simulink model "SF003A_Dampg"  (R2013b)
settings: Solver=FixedStepDiscrete  StartTime=0.0  StopTime=1  FixedStep=.002  RelTol=1e-3
values from neighbouring files (symbols this model uses):
  ARCHGLBPRM_2MILLISEC_SEC_F32 = DataDict.Constant    [SF003A_Dampg_DataDict.m]
  DampgHydBasCoeff1 = DataDict.Calibration    [SF003A_Dampg_DataDict.m]
  DampgHydBasCoeff2 = DataDict.Calibration    [SF003A_Dampg_DataDict.m]
  DampgHydBasCoeff3 = DataDict.Calibration    [SF003A_Dampg_DataDict.m]
  DampgHydBasCoeff4 = DataDict.Calibration    [SF003A_Dampg_DataDict.m]
  DampgHydOutpLim = DataDict.Calibration    [SF003A_Dampg_DataDict.m]
  DampgQuad13Mplr = DataDict.Calibration    [SF003A_Dampg_DataDict.m]
  DampgQuad24Mplr = DataDict.Calibration    [SF003A_Dampg_DataDict.m]
  DampgQuadHwTqBacklsh = DataDict.Calibration    [SF003A_Dampg_DataDict.m]
  DampgQuadMotVelBacklsh = DataDict.Calibration    [SF003A_Dampg_DataDict.m]
  FLTINJ_DAMPG_DAMPGCMDBAS = DataDict.Constant    [SF003A_Dampg_DataDict.m]
libraries: FloatToFixd x9, Fil x8, FixdToFloat x8, LnrIntrpn x7, NxtrAbslt x5, NxtrSign x3, NxtrLim x3, simulink x1, NxtrMax x1, BilnrIntrpnMplX x1
settings Model: Creator=TZ5743  LastModifiedBy=TZ5743
settings DataIOCC: LimitDataPoints=off  SaveFormat=Structure  ReturnWorkspaceOutputs=on
settings OptimizationCC: BlockReduction=off  InlineParams=on  ZeroExternalMemoryAtStartup=off  ZeroInternalMemoryAtStartup=off  OptimizeModelRefInitCode=on  LifeSpan=1
settings DebuggingCC: SignalInfNanChecking=error  SignalRangeChecking=warning  UnderspecifiedInitializationDetection=Simplified  SolverPrmCheckMsg=error  InheritedTsInSrcMsg=error  DiscreteInheritContinuousMsg=error  SingleTaskRateTransMsg=error  TasksWithSamePriorityMsg=error  SigSpecEnsureSampleTimeMsg=error  CheckMatrixSingularityMsg=error  IntegerOverflowMsg=error  ParameterUnderflowMsg=error  ParameterPrecisionLossMsg=error  ParameterTunabilityLossMsg=error  FixptConstUnderflowMsg=warning  FixptConstOverflowMsg=warning  VectorMatrixConversionMsg=error  SignalLabelMismatchMsg=error  UnconnectedInputMsg=error  UnconnectedOutputMsg=error  UnconnectedLineMsg=error  SFcnCompatibilityMsg=error  UniqueDataStoreMsg=warning  BusObjectLabelMismatch=error  RootOutportRequireBusObject=error  AssertControl=DisableAll  ModelReferenceIOMsg=error  ModelReferenceVersionMismatchMessage=warning  ModelReferenceIOMismatchMessage=error  ModelReferenceCSMismatchMessage=warning  ModelReferenceDataLoggingMessage=error  StateNameClashWarn=warning  StrictBusMsg=ErrorOnBusTreatedAsVector  NonBusSignalsTreatedAsBus=error  SFUnexpectedBacktrackingDiag=error  SFInvalidInputDataAccessInChartInitDiag=error  SFNoUnconditionalDefaultTransitionDiag=error  SFTransitionOutsideNaturalParentDiag=error  SFUnconditionalTransitionShadowingDiag=error  SFUndirectedBroadcastEventsDiag=error
settings ModelReferenceCC: ModelReferenceNumInstancesAllowed=Single
settings RTWCC: SystemTargetFile=autosar.tlc  GenCodeOnly=on  TemplateMakefile=ert_default_tmf  Description=AUTOSAR  GenerateReport=on  ProcessScript=autosar_make_rtw_hook  LaunchReport=on
settings CodeAppCC: GenerateComments=off  IgnoreCustomStorageClasses=off  CustomSymbolStrType=$N$R$M  CustomSymbolStrBlkIO=$N$M  SimulinkBlockComments=off
settings STFCustomTargetCC: ParMdlRefBuildCompliant=on  CompOptLevelCompliant=on  IncludeMdlTerminateFcn=off  CombineOutputUpdateFcns=on  SuppressErrorStatus=on  ERTFirstTimeCompliant=on  ERTCustomFileBanners=on  SupportNonFinite=off  SupportComplex=off  SupportContinuousTime=off  SupportNonInlinedSFcns=off  MATLABClassNameForMDSCustomization=Simulink.SoftwareTarget.ERTCustomization  AutosarCompliant=on  GRTInterface=off  SystemTargetFile=autosar.tlc
settings ERTTargetCC: CodeReplacementLibrary=ANSI_C  ConcurrentExecutionCompliant=off  IncludeMdlTerminateFcn=off  SuppressErrorStatus=on  SupportNonFinite=off  SupportComplex=off  ModelStepFunctionPrototypeControlCompliant=off  CPPClassGenCompliant=off  AutosarCompliant=on  InlinedParameterPlacement=NonHierarchical  ERTCustomFileTemplate=example_file_process.tlc  EnableUserReplacementTypes=on

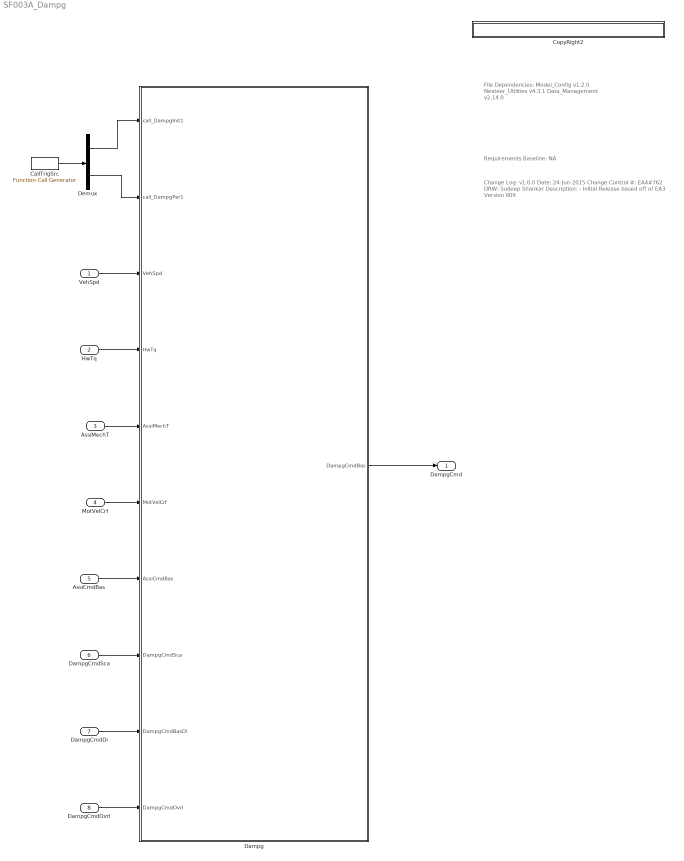
== system SF003A_Dampg ==
  note: File Dependencies:
      |
      | Model_Config v1.2.0
      | Nexteer_Utilities v4.3.1
      | Data_Management v2.14.0
  note: Requirements Baseline: NA
  note: Change Log:
      | v1.0.0
      | Date: 24-Jun-2015
      | Change Control #: EA4#762
      | DRW:  Sudeep Shankar
      | Description:
      | - Initial Release based off of EA3 Version 009
  VehSpd : Inport
  HwTq : Inport  Port=2
  AssiMechT : Inport  Port=3
  MotVelCrf : Inport  Port=4
  AssiCmdBas : Inport  Port=5
  DampgCmdSca : Inport  Port=6
  DampgCmdDi : Inport  Port=7
  DampgCmdOvrl : Inport  Port=8
  CallTrigSrc : simulink/Ports & Subsystems/Function-Call Generator  RequirementInfo={} %GIDa_ba0e12fc_4474_4f55_8217_81b6c7a3534f  sample_time=0.002  numberOfIterations=1
  CopyRight2 : Subsystem  Description=|  mask(Copyright Information){none=on}
      | Copyright info block.                                               
      |                                                                     
      | Place copyright information at the top of every subsystem in design.
      mask prompts: none "No parameters"
      mask help: Place copyright information at the top of every subsystem in design.
      mask Display:
      | NxtrConf = 'Nexteer Confidential';
      | 
      | sys = bdroot; %handle for the current model ("system")
      | first = get_param(sys,'Created');
      | if(isempty(first))
      |     first = datestr(now,'yyyy');
      | else
      |     first = first(end-3:end);  %year is last four digits
      | end
      | 
      | last = get_param(sys,'LastModifiedDate');
      | if isempty(last)
      |     last = datestr(now,'yyyy');
      | else
      |     last = last(end-3:end);
      | end
      | 
      | if strcmp(first,last)
      |     fprintf('%s -- Copyright %s Nexteer',NxtrConf,first)
      | else
      |     fprintf('%s -- %s%s- %s Nexteer',NxtrConf,char(169),first,last)
      | end
  Dampg : Subsystem
  Demux : Demux  Outputs=2
  DampgCmd : Outport
  wires:
  Demux/2 -> Dampg/2(call_DampgPer1)
  VehSpd/1 -> Dampg/3(VehSpd)
  HwTq/1 -> Dampg/4(HwTq)
  AssiMechT/1 -> Dampg/5(AssiMechT)
  MotVelCrf/1 -> Dampg/6(MotVelCrf)
  AssiCmdBas/1 -> Dampg/7(AssiCmdBas)
  DampgCmdSca/1 -> Dampg/8(DampgCmdSca)
  DampgCmdDi/1 -> Dampg/9(DampgCmdBasDi)
  DampgCmdOvrl/1 -> Dampg/10(DampgCmdOvrl)
  Dampg/1(DampgCmdBas) -> DampgCmd/1
  CallTrigSrc/1 -> Demux/1
  Demux/1 -> Dampg/1(call_DampgInit1)

== system SF003A_Dampg/CopyRight2 ==

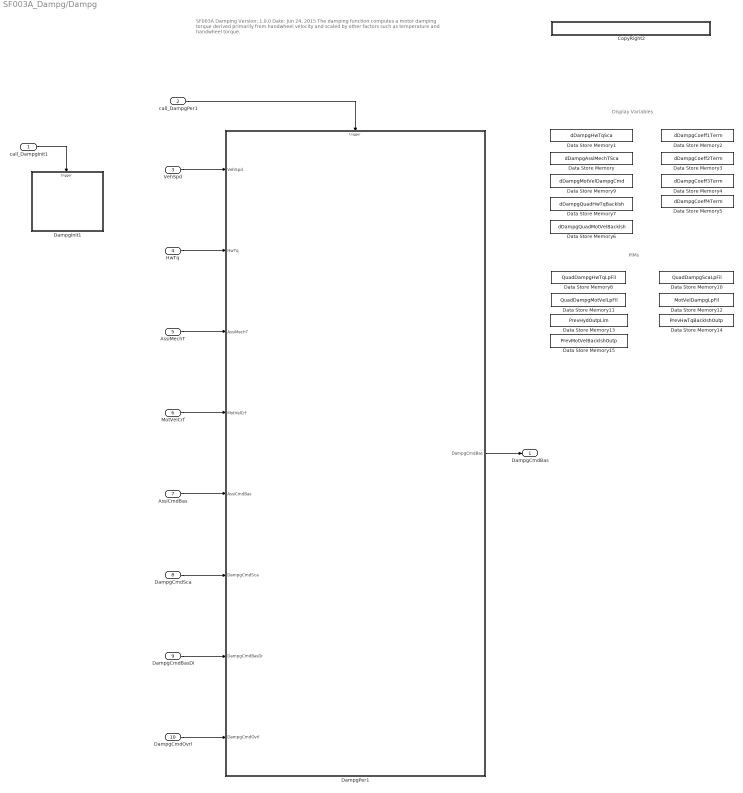
== system SF003A_Dampg/Dampg ==
  note: PIMs
  note: Display Variables
  note: SF003A Damping       Version: 1.0.0                                                      Date:  Jun 24, 2015
      |
      | The damping function computes a motor damping torque derived primarily from handwheel velocity and scaled by
      | other factors such as temperature and handwheel torque.
  call_DampgInit1 : Inport
  call_DampgPer1 : Inport  Port=2
  VehSpd : Inport  Port=3
  HwTq : Inport  Port=4
  AssiMechT : Inport  Port=5
  MotVelCrf : Inport  Port=6
  AssiCmdBas : Inport  Port=7
  DampgCmdSca : Inport  Port=8
  DampgCmdBasDi : Inport  Port=9
  DampgCmdOvrl : Inport  Port=10
  CopyRight2 : Subsystem  Description=|  mask(Copyright Information){none=on}
      | Copyright info block.                                               
      |                                                                     
      | Place copyright information at the top of every subsystem in design.
      mask prompts: none "No parameters"
      mask help: Place copyright information at the top of every subsystem in design.
      mask Display:
      | NxtrConf = 'Nexteer Confidential';
      | 
      | sys = bdroot; %handle for the current model ("system")
      | first = get_param(sys,'Created');
      | if(isempty(first))
      |     first = datestr(now,'yyyy');
      | else
      |     first = first(end-3:end);  %year is last four digits
      | end
      | 
      | last = get_param(sys,'LastModifiedDate');
      | if isempty(last)
      |     last = datestr(now,'yyyy');
      | else
      |     last = last(end-3:end);
      | end
      | 
      | if strcmp(first,last)
      |     fprintf('%s -- Copyright %s Nexteer',NxtrConf,first)
      | else
      |     fprintf('%s -- %s%s- %s Nexteer',NxtrConf,char(169),first,last)
      | end
  DampgInit1 : Subsystem
  DampgPer1 : Subsystem
  Data Store Memory : DataStoreMemory  DataStoreName=dDampgAssiMechTSca  ReadBeforeWriteMsg=warning  WriteAfterWriteMsg=warning  WriteAfterReadMsg=warning  StateMustResolveToSignalObject=on
  Data Store Memory1 : DataStoreMemory  DataStoreName=dDampgHwTqSca  ReadBeforeWriteMsg=warning  WriteAfterWriteMsg=warning  WriteAfterReadMsg=warning  OutDataTypeStr=single  StateMustResolveToSignalObject=on
  Data Store Memory10 : DataStoreMemory  DataStoreName=QuadDampgScaLpFil  InitialValue=struct('FilSt',single(0),'FilGain',single(0))  OutDataTypeStr=Bus: FilLpRec1  StateMustResolveToSignalObject=on
  Data Store Memory11 : DataStoreMemory  DataStoreName=QuadDampgMotVelLpFil  InitialValue=struct('FilSt',single(0),'FilGain',single(0))  OutDataTypeStr=Bus: FilLpRec1  StateMustResolveToSignalObject=on
  Data Store Memory12 : DataStoreMemory  DataStoreName=MotVelDampgLpFil  InitialValue=struct('FilSt',single(0),'FilGain',single(0))  OutDataTypeStr=Bus: FilLpRec1  StateMustResolveToSignalObject=on
  Data Store Memory13 : DataStoreMemory  DataStoreName=PrevHydOutpLim  StateMustResolveToSignalObject=on
  Data Store Memory14 : DataStoreMemory  DataStoreName=PrevHwTqBacklshOutp  StateMustResolveToSignalObject=on
  Data Store Memory15 : DataStoreMemory  DataStoreName=PrevMotVelBacklshOutp  StateMustResolveToSignalObject=on
  Data Store Memory2 : DataStoreMemory  DataStoreName=dDampgCoeff1Term  ReadBeforeWriteMsg=warning  WriteAfterWriteMsg=warning  WriteAfterReadMsg=warning  OutDataTypeStr=single  StateMustResolveToSignalObject=on
  Data Store Memory3 : DataStoreMemory  DataStoreName=dDampgCoeff2Term  ReadBeforeWriteMsg=warning  WriteAfterWriteMsg=warning  WriteAfterReadMsg=warning  OutDataTypeStr=single  StateMustResolveToSignalObject=on
  Data Store Memory4 : DataStoreMemory  DataStoreName=dDampgCoeff3Term  ReadBeforeWriteMsg=warning  WriteAfterWriteMsg=warning  WriteAfterReadMsg=warning  OutDataTypeStr=single  StateMustResolveToSignalObject=on
  Data Store Memory5 : DataStoreMemory  DataStoreName=dDampgCoeff4Term  ReadBeforeWriteMsg=warning  WriteAfterWriteMsg=warning  WriteAfterReadMsg=warning  OutDataTypeStr=single  StateMustResolveToSignalObject=on
  Data Store Memory6 : DataStoreMemory  DataStoreName=dDampgQuadMotVelBacklsh  ReadBeforeWriteMsg=warning  WriteAfterWriteMsg=warning  WriteAfterReadMsg=warning  StateMustResolveToSignalObject=on
  Data Store Memory7 : DataStoreMemory  DataStoreName=dDampgQuadHwTqBacklsh  ReadBeforeWriteMsg=warning  WriteAfterWriteMsg=warning  WriteAfterReadMsg=warning  StateMustResolveToSignalObject=on
  Data Store Memory8 : DataStoreMemory  DataStoreName=QuadDampgHwTqLpFil  InitialValue=struct('FilSt',single(0),'FilGain',single(0))  OutDataTypeStr=Bus: FilLpRec1  StateMustResolveToSignalObject=on
  Data Store Memory9 : DataStoreMemory  DataStoreName=dDampgMotVelDampgCmd  ReadBeforeWriteMsg=warning  WriteAfterWriteMsg=warning  WriteAfterReadMsg=warning  StateMustResolveToSignalObject=on
  DampgCmdBas : Outport
  wires:
  MotVelCrf/1 -> DampgPer1/4(MotVelCrf)
  DampgCmdBasDi/1 -> DampgPer1/7(DampgCmdBasDi)
  DampgPer1/1(DampgCmdBas) -> DampgCmdBas/1
  DampgCmdSca/1 -> DampgPer1/6(DampgCmdSca)
  AssiMechT/1 -> DampgPer1/3(AssiMechT)
  DampgCmdOvrl/1 -> DampgPer1/8(DampgCmdOvrl)
  HwTq/1 -> DampgPer1/2(HwTq)
  AssiCmdBas/1 -> DampgPer1/5(AssiCmdBas)
  VehSpd/1 -> DampgPer1/1(VehSpd)
  call_DampgPer1/1 -> DampgPer1/Trigger
  call_DampgInit1/1 -> DampgInit1/Trigger

== system SF003A_Dampg/Dampg/CopyRight2 ==

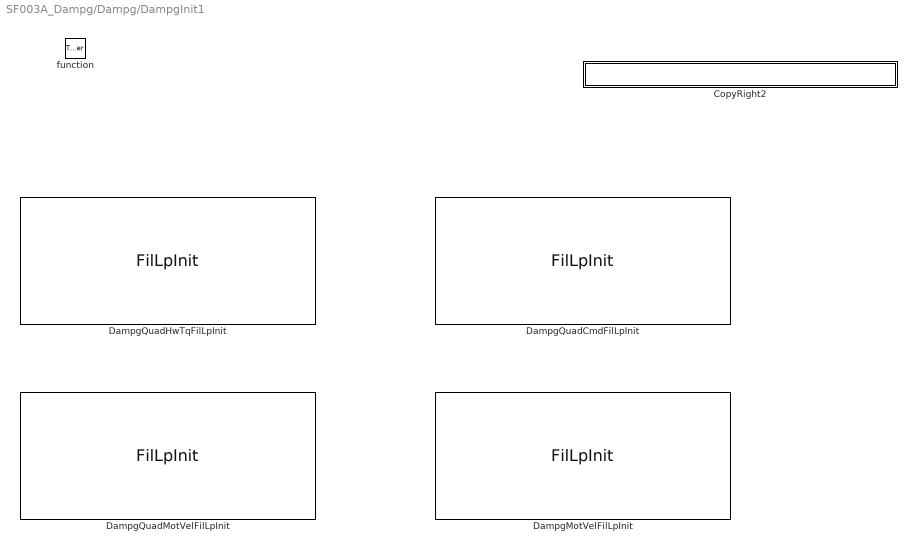
== system SF003A_Dampg/Dampg/DampgInit1 ==
  function : TriggerPort  TriggerType=function-call
  CopyRight2 : Subsystem  Description=|  mask(Copyright Information){none=on}
      | Copyright info block.                                               
      |                                                                     
      | Place copyright information at the top of every subsystem in design.
      mask prompts: none "No parameters"
      mask help: Place copyright information at the top of every subsystem in design.
      mask Display:
      | NxtrConf = 'Nexteer Confidential';
      | 
      | sys = bdroot; %handle for the current model ("system")
      | first = get_param(sys,'Created');
      | if(isempty(first))
      |     first = datestr(now,'yyyy');
      | else
      |     first = first(end-3:end);  %year is last four digits
      | end
      | 
      | last = get_param(sys,'LastModifiedDate');
      | if isempty(last)
      |     last = datestr(now,'yyyy');
      | else
      |     last = last(end-3:end);
      | end
      | 
      | if strcmp(first,last)
      |     fprintf('%s -- Copyright %s Nexteer',NxtrConf,first)
      | else
      |     fprintf('%s -- %s%s- %s Nexteer',NxtrConf,char(169),first,last)
      | end
  DampgMotVelFilLpInit : Fil/FilLpInit  Ic=0  Ts=ARCHGLBPRM_2MILLISEC_SEC_F32  Freq=DampgMotVelLpFilFrq  StVar=MotVelDampgLpFil
  DampgQuadCmdFilLpInit : Fil/FilLpInit  Ic=0  Ts=ARCHGLBPRM_2MILLISEC_SEC_F32  Freq=DampgQuadScaLpFilFrq  StVar=QuadDampgScaLpFil
  DampgQuadHwTqFilLpInit : Fil/FilLpInit  Ic=0  Ts=ARCHGLBPRM_2MILLISEC_SEC_F32  Freq=DampgQuadHwTqLpFilFrq  StVar=QuadDampgHwTqLpFil
  DampgQuadMotVelFilLpInit : Fil/FilLpInit  Ic=0  Ts=ARCHGLBPRM_2MILLISEC_SEC_F32  Freq=DampgQuadMotVelLpFilFrq  StVar=QuadDampgMotVelLpFil

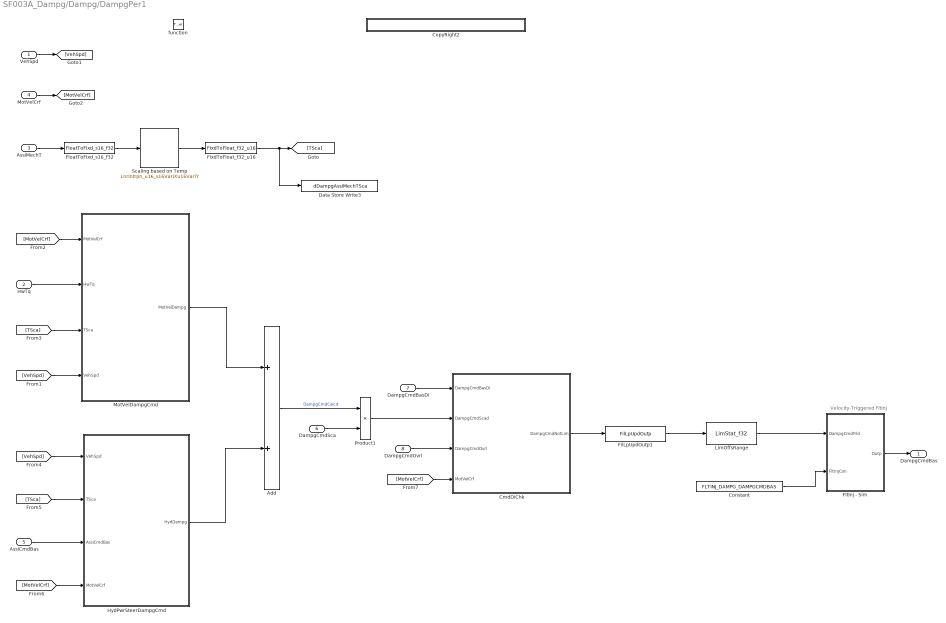
== system SF003A_Dampg/Dampg/DampgPer1 ==
  note: Velocity-Triggered FltInj
  VehSpd : Inport
  HwTq : Inport  Port=2
  AssiMechT : Inport  Port=3
  MotVelCrf : Inport  Port=4
  AssiCmdBas : Inport  Port=5
  DampgCmdSca : Inport  Port=6
  DampgCmdBasDi : Inport  Port=7
  DampgCmdOvrl : Inport  Port=8
  function : TriggerPort  TriggerType=function-call
  Add : Sum
  CmdDiChk : Subsystem
  Constant : Constant  Value=FLTINJ_DAMPG_DAMPGCMDBAS
  CopyRight2 : Subsystem  Description=|  mask(Copyright Information){none=on}
      | Copyright info block.                                               
      |                                                                     
      | Place copyright information at the top of every subsystem in design.
      mask prompts: none "No parameters"
      mask help: Place copyright information at the top of every subsystem in design.
      mask Display:
      | NxtrConf = 'Nexteer Confidential';
      | 
      | sys = bdroot; %handle for the current model ("system")
      | first = get_param(sys,'Created');
      | if(isempty(first))
      |     first = datestr(now,'yyyy');
      | else
      |     first = first(end-3:end);  %year is last four digits
      | end
      | 
      | last = get_param(sys,'LastModifiedDate');
      | if isempty(last)
      |     last = datestr(now,'yyyy');
      | else
      |     last = last(end-3:end);
      | end
      | 
      | if strcmp(first,last)
      |     fprintf('%s -- Copyright %s Nexteer',NxtrConf,first)
      | else
      |     fprintf('%s -- %s%s- %s Nexteer',NxtrConf,char(169),first,last)
      | end
  Data Store Write3 : DataStoreWrite  DataStoreName=dDampgAssiMechTSca
  FilLpUpdOutp1 : Fil/FilLpUpdOutp  StVar=MotVelDampgLpFil
      settings: AttributesFormatString=StVar: %<StVar>
  FixdToFloat_f32_u16 : FixdToFloat/FixdToFloat_f32_u16  Param1=12
  FloatToFixd_s16_f32 : FloatToFixd/FloatToFixd_s16_f32  Param1=7
  FltInj - Sim : Subsystem  TreatAsAtomicUnit=on  VariantControl=FltInj_sim  mask(Fault_Injection){}
      mask help: Fault Injection is a simulation only block for EA4 programs.
  HydPwrSteerDampgCmd : Subsystem
  LimOffsRange : NxtrLim/LimStat_f32  LoLim=SYSGLBPRM_MOTTQCMDLOLIM_MOTNWTMTR_F32  HiLim=SYSGLBPRM_MOTTQCMDHILIM_MOTNWTMTR_F32
      settings: AttributesFormatString=|
      | Low Limit: %<LoLim>
      | High Limit:%<HiLim>
  MotVelDampgCmd : Subsystem
  Product1 : Product  RndMeth=Zero
  Scaling based on Temp : LnrIntrpn/LnrIntrpn_u16_s16VariXu16VariY  XTbl=DampgTScaX  YTbl=DampgTScaY
      settings: AttributesFormatString=Lnr ( s16VariX , u16VariY )
  DampgCmdBas : Outport
  wires:
  Constant/1 -> FltInj - Sim/2(FltInjCon)
  FltInj - Sim/1(Outp) -> DampgCmdBas/1
  Product1/1 -> CmdDiChk/2(DampgCmdScad)
  CmdDiChk/1(DampgCmdNotLim) -> FilLpUpdOutp1/1
  DampgCmdOvrl/1 -> CmdDiChk/3(DampgCmdOvrl)
  DampgCmdBasDi/1 -> CmdDiChk/1(DampgCmdBasDi)
  LimOffsRange/1 -> FltInj - Sim/1(DampgCmdFild)
  Scaling based on Temp/1 -> FixdToFloat_f32_u16/1
  AssiMechT/1 -> FloatToFixd_s16_f32/1
  FloatToFixd_s16_f32/1 -> Scaling based on Temp/1
  FixdToFloat_f32_u16/1 -> Data Store Write3/1, [TSca]
  VehSpd/1 -> [VehSpd]
  MotVelCrf/1 -> [MotVelCrf]
  HwTq/1 -> MotVelDampgCmd/2(HwTq)
  [MotVelCrf] -> MotVelDampgCmd/1(MotVelCrf)
  [VehSpd] -> MotVelDampgCmd/4(VehSpd)
  [TSca] -> MotVelDampgCmd/3(TSca)
  [VehSpd] -> HydPwrSteerDampgCmd/1(VehSpd)
  [TSca] -> HydPwrSteerDampgCmd/2(TSca)
  AssiCmdBas/1 -> HydPwrSteerDampgCmd/3(AssiCmdBas)
  [MotVelCrf] -> HydPwrSteerDampgCmd/4(MotVelCrf)
  HydPwrSteerDampgCmd/1(HydDampg) -> Add/2
  MotVelDampgCmd/1(MotVelDampg) -> Add/1
  Add/1 -> Product1/1  "DampgCmdCalcd"
  DampgCmdSca/1 -> Product1/2
  [MotVelCrf] -> CmdDiChk/4(MotVelCrf)
  FilLpUpdOutp1/1 -> LimOffsRange/1

== system SF003A_Dampg/Dampg/DampgInit1/CopyRight2 ==

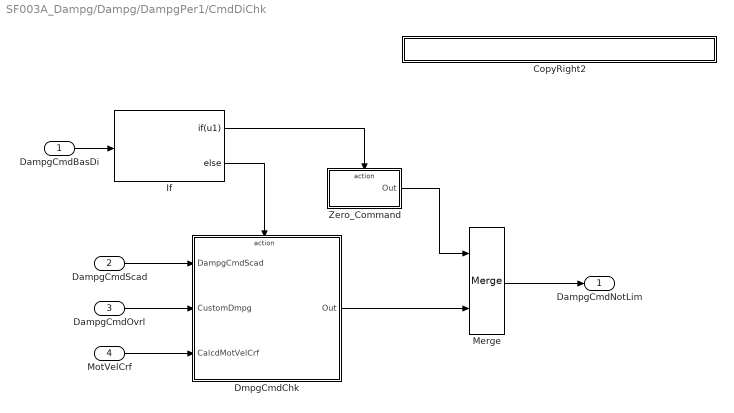
== system SF003A_Dampg/Dampg/DampgPer1/CmdDiChk ==
  DampgCmdBasDi : Inport
  DampgCmdScad : Inport  Port=2
  DampgCmdOvrl : Inport  Port=3
  MotVelCrf : Inport  Port=4
  CopyRight2 : Subsystem  Description=|  mask(Copyright Information){none=on}
      | Copyright info block.                                               
      |                                                                     
      | Place copyright information at the top of every subsystem in design.
      mask prompts: none "No parameters"
      mask help: Place copyright information at the top of every subsystem in design.
      mask Display:
      | NxtrConf = 'Nexteer Confidential';
      | 
      | sys = bdroot; %handle for the current model ("system")
      | first = get_param(sys,'Created');
      | if(isempty(first))
      |     first = datestr(now,'yyyy');
      | else
      |     first = first(end-3:end);  %year is last four digits
      | end
      | 
      | last = get_param(sys,'LastModifiedDate');
      | if isempty(last)
      |     last = datestr(now,'yyyy');
      | else
      |     last = last(end-3:end);
      | end
      | 
      | if strcmp(first,last)
      |     fprintf('%s -- Copyright %s Nexteer',NxtrConf,first)
      | else
      |     fprintf('%s -- %s%s- %s Nexteer',NxtrConf,char(169),first,last)
      | end
  DmpgCmdChk : Subsystem  RequirementInfo={} %GIDa_42609f80_721e_4222_a854_978db5b32e82  TreatAsAtomicUnit=on
  If : If  RequirementInfo={} %GIDa_e8daf89a_735d_4ce3_8883_6d943d5da402  IfExpression=u1
  Merge : Merge
  Zero_Command : Subsystem  RequirementInfo={} %GIDa_8150363f_e871_4e58_837a_c9fd5c39bb6f  TreatAsAtomicUnit=on
  DampgCmdNotLim : Outport
  wires:
  If/2 -> DmpgCmdChk/Action
  If/1 -> Zero_Command/Action
  DampgCmdScad/1 -> DmpgCmdChk/1(DampgCmdScad)
  DmpgCmdChk/1(Out) -> Merge/2
  Zero_Command/1(Out) -> Merge/1
  Merge/1 -> DampgCmdNotLim/1
  DampgCmdBasDi/1 -> If/1
  DampgCmdOvrl/1 -> DmpgCmdChk/2(CustomDmpg)
  MotVelCrf/1 -> DmpgCmdChk/3(CalcdMotVelCrf)

== system SF003A_Dampg/Dampg/DampgPer1/CopyRight2 ==

== system SF003A_Dampg/Dampg/DampgPer1/FltInj - Sim ==
  note: Inport #2 must be Constant
  note: EA4.x Fault Injection
  note: This block requires no modification by FDD author.
      |
      | This block does not actually simulate any fault injection.  It is simply a pass-thru.
      |
      | The port (#2) simply terminates its signal, but we are trying to force the FDD author
      | to properly use the Constant in FDD model.
  DampgCmdFild : Inport
  FltInjCon : Inport  Port=2
  CopyRight2 : Subsystem  Description=|  mask(Copyright Information){none=on}
      | Copyright info block.                                               
      |                                                                     
      | Place copyright information at the top of every subsystem in design.
      mask prompts: none "No parameters"
      mask help: Place copyright information at the top of every subsystem in design.
      mask Display:
      | NxtrConf = 'Nexteer Confidential';
      | 
      | sys = bdroot; %handle for the current model ("system")
      | first = get_param(sys,'Created');
      | if(isempty(first))
      |     first = datestr(now,'yyyy');
      | else
      |     first = first(end-3:end);  %year is last four digits
      | end
      | 
      | last = get_param(sys,'LastModifiedDate');
      | if isempty(last)
      |     last = datestr(now,'yyyy');
      | else
      |     last = last(end-3:end);
      | end
      | 
      | if strcmp(first,last)
      |     fprintf('%s -- Copyright %s Nexteer',NxtrConf,first)
      | else
      |     fprintf('%s -- %s%s- %s Nexteer',NxtrConf,char(169),first,last)
      | end
  Terminator : Terminator
  Outp : Outport
  wires:
  FltInjCon/1 -> Terminator/1
  DampgCmdFild/1 -> Outp/1

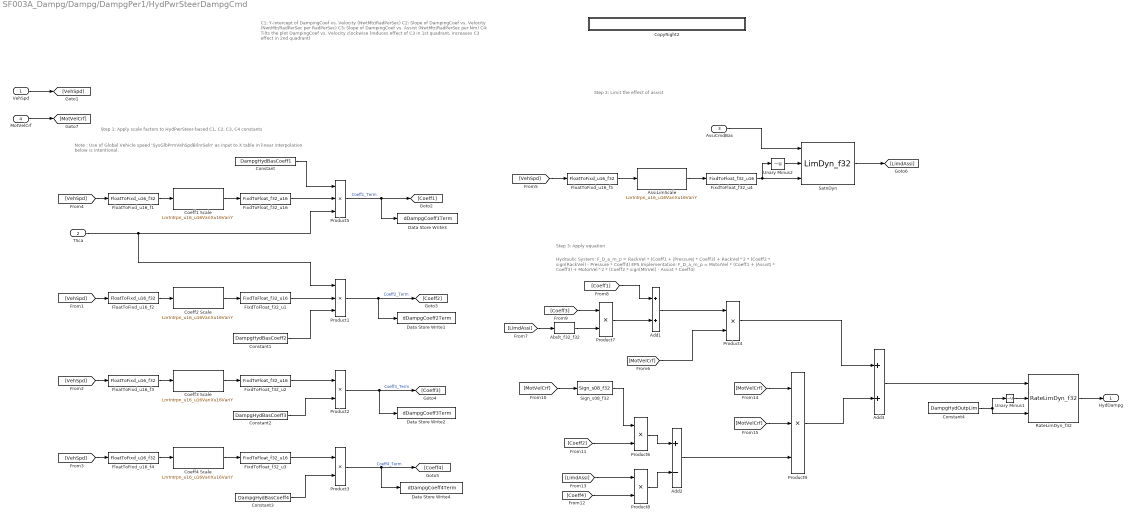
== system SF003A_Dampg/Dampg/DampgPer1/HydPwrSteerDampgCmd ==
  note: Note : Use of Global Vehicle speed 'SysGlbPrmVehSpdBilnrSeln' as input to X table in linear interpolation below is intentional.
  note: Hydraulic System:  F_D_a_m_p = RackVel * (Coeff1 + |Pressure| * Coeff3) + RackVel^2 * (Coeff2 * sign(RackVel) - Pressure * Coeff4)
      | EPS Implementation:  F_D_a_m_p = MotorVel * (Coeff1 + |Assist| * Coeff3) + MotorVel^2 * (Coeff2 * sign(MtrVel) - Assist * Coeff4)
  note: Step 3: Apply equation
  note: Step 2: Limit the effect of assist
  note: C1:  Y-intercept of DampingCoef vs. Velocity  (NwtMtr/RadPerSec)
      | C2:  Slope         of DampingCoef vs. Velocity  (NwtMtr/RadPerSec per RadPerSec)
      |
      | C3:  Slope         of DampingCoef vs. Assist      (NwtMtr/RadPerSec per Nm)
      | C4:  Tilts the plot   DampingCoef vs. Velocity clockwise (reduces effect of C3 in 1st quadrant, increases C3 effect in 2nd quadrant)
  note: Step 1: Apply scale factors to HydPwrSteer-based C1, C2, C3, C4 constants
  VehSpd : Inport
  TSca : Inport  Port=2
  AssiCmdBas : Inport  Port=3
  MotVelCrf : Inport  Port=4
  Abslt_f32_f32 : NxtrAbslt/Abslt_f32_f32  SFunctionSpec=single y1 = Abslt_f32_f32(single u1)
      settings: AttributesFormatString=%<Name>
  Add1 : Sum
  Add2 : Sum  Inputs=+-
  Add3 : Sum
  AssiLimScale : LnrIntrpn/LnrIntrpn_u16_u16VariXu16VariY  XTbl=SysGlbPrmVehSpdBilnrSeln  YTbl=DampgHydAssiLim
      settings: AttributesFormatString=Lnr ( u16VariX , u16VariY )
  Coeff1 Scale : LnrIntrpn/LnrIntrpn_u16_u16VariXu16VariY  XTbl=SysGlbPrmVehSpdBilnrSeln  YTbl=DampgHydCoeff1ScaY
      settings: AttributesFormatString=Lnr ( u16VariX , u16VariY )
  Coeff2 Scale : LnrIntrpn/LnrIntrpn_u16_u16VariXu16VariY  XTbl=SysGlbPrmVehSpdBilnrSeln  YTbl=DampgHydCoeff2ScaY
      settings: AttributesFormatString=Lnr ( u16VariX , u16VariY )
  Coeff3 Scale : LnrIntrpn/LnrIntrpn_u16_u16VariXu16VariY  XTbl=SysGlbPrmVehSpdBilnrSeln  YTbl=DampgHydCoeff3ScaY
      settings: AttributesFormatString=Lnr ( u16VariX , u16VariY )
  Coeff4 Scale : LnrIntrpn/LnrIntrpn_u16_u16VariXu16VariY  XTbl=SysGlbPrmVehSpdBilnrSeln  YTbl=DampgHydCoeff4ScaY
      settings: AttributesFormatString=Lnr ( u16VariX , u16VariY )
  Constant : Constant  Value=DampgHydBasCoeff1
  Constant1 : Constant  Value=DampgHydBasCoeff2
  Constant2 : Constant  Value=DampgHydBasCoeff3
  Constant3 : Constant  Value=DampgHydBasCoeff4
  Constant4 : Constant  Value=DampgHydOutpLim
  CopyRight2 : Subsystem  Description=|  mask(Copyright Information){none=on}
      | Copyright info block.                                               
      |                                                                     
      | Place copyright information at the top of every subsystem in design.
      mask prompts: none "No parameters"
      mask help: Place copyright information at the top of every subsystem in design.
      mask Display:
      | NxtrConf = 'Nexteer Confidential';
      | 
      | sys = bdroot; %handle for the current model ("system")
      | first = get_param(sys,'Created');
      | if(isempty(first))
      |     first = datestr(now,'yyyy');
      | else
      |     first = first(end-3:end);  %year is last four digits
      | end
      | 
      | last = get_param(sys,'LastModifiedDate');
      | if isempty(last)
      |     last = datestr(now,'yyyy');
      | else
      |     last = last(end-3:end);
      | end
      | 
      | if strcmp(first,last)
      |     fprintf('%s -- Copyright %s Nexteer',NxtrConf,first)
      | else
      |     fprintf('%s -- %s%s- %s Nexteer',NxtrConf,char(169),first,last)
      | end
  Data Store Write1 : DataStoreWrite  DataStoreName=dDampgCoeff2Term
  Data Store Write2 : DataStoreWrite  DataStoreName=dDampgCoeff3Term
  Data Store Write3 : DataStoreWrite  DataStoreName=dDampgCoeff1Term
  Data Store Write4 : DataStoreWrite  DataStoreName=dDampgCoeff4Term
  FixdToFloat_f32_u{1..4,16} (5 alike) : FixdToFloat/FixdToFloat_f32_u16  Param1=12
  FloatToFixd_u16_f{1..5} (5 alike) : FloatToFixd/FloatToFixd_u16_f32  Param1=7
  Product1 : Product  Inputs=3  RndMeth=Zero
  Product{2..4,6..8} (6 alike) : Product  RndMeth=Zero
  Product5 : Product  Inputs=3  RndMeth=Zero
  Product9 : Product  Inputs=3  RndMeth=Zero
  RateLimDyn_f32 : NxtrLim/RateLimDyn_f32  StVar=PrevHydOutpLim  Ts=ARCHGLBPRM_2MILLISEC_SEC_F32
      settings: AttributesFormatString=StVar: %<StVar>
  SatnDyn : NxtrLim/LimDyn_f32
  Sign_s08_f32 : NxtrSign/Sign_s08_f32  SFunctionSpec=int8 y1 = Sign_s08_f32(single u1)
  Unary Minus1 : UnaryMinus
  Unary Minus2 : UnaryMinus
  HydDampg : Outport
  wires:
  FloatToFixd_u16_f1/1 -> Coeff1 Scale/1
  Coeff1 Scale/1 -> FixdToFloat_f32_u16/1
  Constant/1 -> Product5/1
  TSca/1 -> Product5/3, Product1/1
  FixdToFloat_f32_u16/1 -> Product5/2
  Product5/1 -> Data Store Write3/1, [Coeff1]  "Coeff1_Term"
  VehSpd/1 -> [VehSpd]
  [VehSpd] -> FloatToFixd_u16_f1/1
  FloatToFixd_u16_f2/1 -> Coeff2 Scale/1
  Coeff2 Scale/1 -> FixdToFloat_f32_u1/1
  FixdToFloat_f32_u1/1 -> Product1/2
  Product1/1 -> Data Store Write1/1, [Coeff2]  "Coeff2_Term"
  [VehSpd] -> FloatToFixd_u16_f2/1
  Constant1/1 -> Product1/3
  FloatToFixd_u16_f3/1 -> Coeff3 Scale/1
  Coeff3 Scale/1 -> FixdToFloat_f32_u2/1
  FixdToFloat_f32_u2/1 -> Product2/1
  [VehSpd] -> FloatToFixd_u16_f3/1
  Constant2/1 -> Product2/2
  Product2/1 -> Data Store Write2/1, [Coeff3]  "Coeff3_Term"
  FloatToFixd_u16_f4/1 -> Coeff4 Scale/1
  Coeff4 Scale/1 -> FixdToFloat_f32_u3/1
  FixdToFloat_f32_u3/1 -> Product3/1
  [VehSpd] -> FloatToFixd_u16_f4/1
  Constant3/1 -> Product3/2
  Product3/1 -> Data Store Write4/1, [Coeff4]  "Coeff4_Term"
  [VehSpd] -> FloatToFixd_u16_f5/1
  FloatToFixd_u16_f5/1 -> AssiLimScale/1
  AssiCmdBas/1 -> SatnDyn/1
  AssiLimScale/1 -> FixdToFloat_f32_u4/1
  Unary Minus2/1 -> SatnDyn/2
  FixdToFloat_f32_u4/1 -> Unary Minus2/1, SatnDyn/3
  SatnDyn/1 -> [LimdAssi]
  MotVelCrf/1 -> [MotVelCrf]
  [MotVelCrf] -> Product4/2
  Product7/1 -> Add1/2
  [Coeff1] -> Add1/1
  [Coeff3] -> Product7/1
  [LimdAssi] -> Abslt_f32_f32/1
  Abslt_f32_f32/1 -> Product7/2
  Add1/1 -> Product4/1
  [MotVelCrf] -> Sign_s08_f32/1
  Sign_s08_f32/1 -> Product6/1
  [Coeff2] -> Product6/2
  [LimdAssi] -> Product8/1
  [Coeff4] -> Product8/2
  Product8/1 -> Add2/2
  Product6/1 -> Add2/1
  Add2/1 -> Product9/3
  [MotVelCrf] -> Product9/1
  [MotVelCrf] -> Product9/2
  Product4/1 -> Add3/1
  Product9/1 -> Add3/2
  Add3/1 -> RateLimDyn_f32/1
  RateLimDyn_f32/1 -> HydDampg/1
  Constant4/1 -> Unary Minus1/1, RateLimDyn_f32/3
  Unary Minus1/1 -> RateLimDyn_f32/2

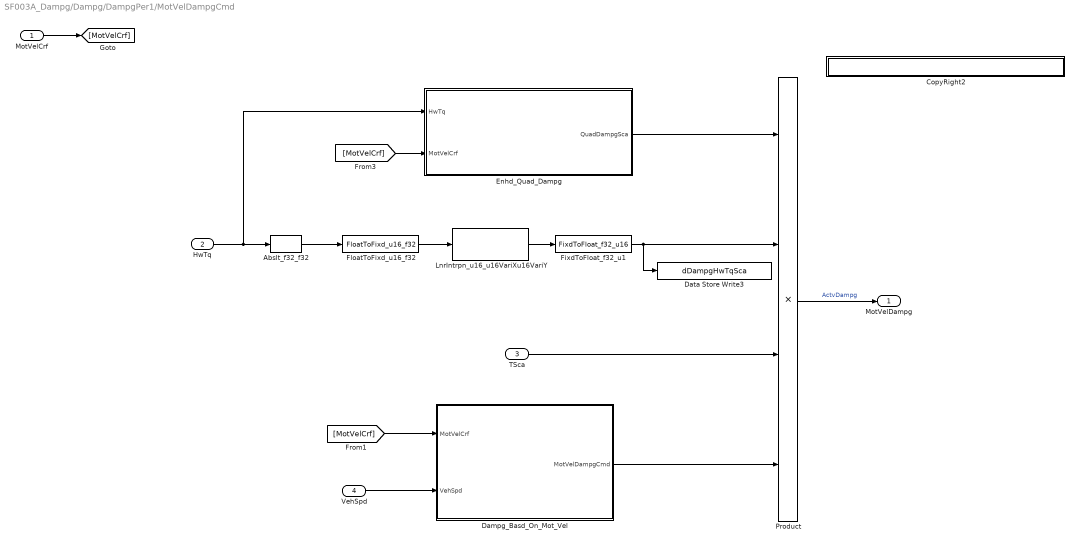
== system SF003A_Dampg/Dampg/DampgPer1/MotVelDampgCmd ==
  MotVelCrf : Inport
  HwTq : Inport  Port=2
  TSca : Inport  Port=3
  VehSpd : Inport  Port=4
  Abslt_f32_f32 : NxtrAbslt/Abslt_f32_f32  SFunctionSpec=single y1 = Abslt_f32_f32(single u1)
      settings: AttributesFormatString=%<Name>
  CopyRight2 : Subsystem  Description=|  mask(Copyright Information){none=on}
      | Copyright info block.                                               
      |                                                                     
      | Place copyright information at the top of every subsystem in design.
      mask prompts: none "No parameters"
      mask help: Place copyright information at the top of every subsystem in design.
      mask Display:
      | NxtrConf = 'Nexteer Confidential';
      | 
      | sys = bdroot; %handle for the current model ("system")
      | first = get_param(sys,'Created');
      | if(isempty(first))
      |     first = datestr(now,'yyyy');
      | else
      |     first = first(end-3:end);  %year is last four digits
      | end
      | 
      | last = get_param(sys,'LastModifiedDate');
      | if isempty(last)
      |     last = datestr(now,'yyyy');
      | else
      |     last = last(end-3:end);
      | end
      | 
      | if strcmp(first,last)
      |     fprintf('%s -- Copyright %s Nexteer',NxtrConf,first)
      | else
      |     fprintf('%s -- %s%s- %s Nexteer',NxtrConf,char(169),first,last)
      | end
  Dampg_Basd_On_Mot_Vel : Subsystem
  Data Store Write3 : DataStoreWrite  DataStoreName=dDampgHwTqSca
  "Enhd_Quad_Dampg " : Subsystem
  FixdToFloat_f32_u1 : FixdToFloat/FixdToFloat_f32_u16  Param1=15
  FloatToFixd_u16_f32 : FloatToFixd/FloatToFixd_u16_f32  Param1=8
  LnrIntrpn_u16_u16VariXu16VariY : LnrIntrpn/LnrIntrpn_u16_u16VariXu16VariY  XTbl=DampgHwTqX  YTbl=DampgHwTqY
      settings: AttributesFormatString=Lnr ( u16VariX , u16VariY )
  Product : Product  Inputs=4  RndMeth=Zero
  MotVelDampg : Outport
  wires:
  HwTq/1 -> Abslt_f32_f32/1, "Enhd_Quad_Dampg "/1(HwTq)
  FloatToFixd_u16_f32/1 -> LnrIntrpn_u16_u16VariXu16VariY/1
  LnrIntrpn_u16_u16VariXu16VariY/1 -> FixdToFloat_f32_u1/1
  Dampg_Basd_On_Mot_Vel/1(MotVelDampgCmd) -> Product/4
  FixdToFloat_f32_u1/1 -> Product/2, Data Store Write3/1
  Abslt_f32_f32/1 -> FloatToFixd_u16_f32/1
  "Enhd_Quad_Dampg "/1(QuadDampgSca) -> Product/1
  Product/1 -> MotVelDampg/1  "ActvDampg"
  TSca/1 -> Product/3
  MotVelCrf/1 -> [MotVelCrf]
  [MotVelCrf] -> "Enhd_Quad_Dampg "/2(MotVelCrf)
  [MotVelCrf] -> Dampg_Basd_On_Mot_Vel/1(MotVelCrf)
  VehSpd/1 -> Dampg_Basd_On_Mot_Vel/2(VehSpd)

== system SF003A_Dampg/Dampg/DampgPer1/CmdDiChk/CopyRight2 ==

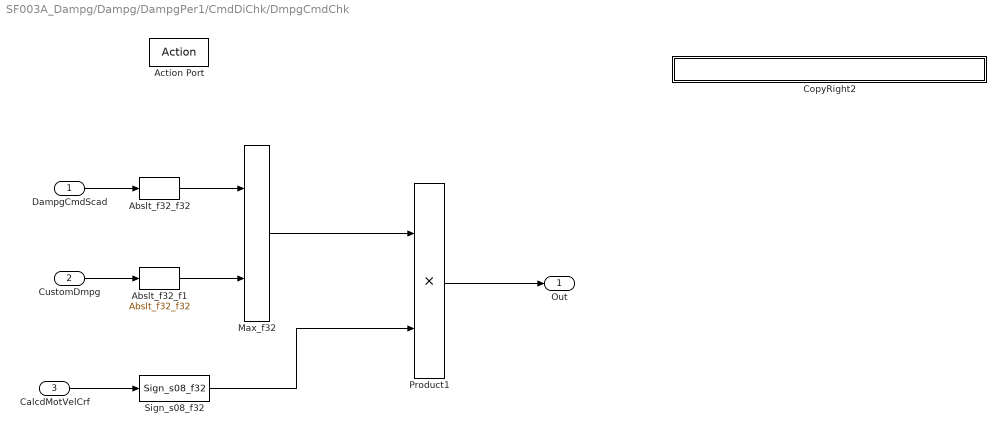
== system SF003A_Dampg/Dampg/DampgPer1/CmdDiChk/DmpgCmdChk ==
  DampgCmdScad : Inport
  CustomDmpg : Inport  Port=2
  CalcdMotVelCrf : Inport  Port=3
  Action Port : ActionPort  ActionType=else
  Abslt_f32_f1 : NxtrAbslt/Abslt_f32_f32  SFunctionSpec=single y1 = Abslt_f32_f32(single u1)
      settings: AttributesFormatString=%<Name>
  Abslt_f32_f32 : NxtrAbslt/Abslt_f32_f32  SFunctionSpec=single y1 = Abslt_f32_f32(single u1)
      settings: AttributesFormatString=%<Name>
  CopyRight2 : Subsystem  Description=|  mask(Copyright Information){none=on}
      | Copyright info block.                                               
      |                                                                     
      | Place copyright information at the top of every subsystem in design.
      mask prompts: none "No parameters"
      mask help: Place copyright information at the top of every subsystem in design.
      mask Display:
      | NxtrConf = 'Nexteer Confidential';
      | 
      | sys = bdroot; %handle for the current model ("system")
      | first = get_param(sys,'Created');
      | if(isempty(first))
      |     first = datestr(now,'yyyy');
      | else
      |     first = first(end-3:end);  %year is last four digits
      | end
      | 
      | last = get_param(sys,'LastModifiedDate');
      | if isempty(last)
      |     last = datestr(now,'yyyy');
      | else
      |     last = last(end-3:end);
      | end
      | 
      | if strcmp(first,last)
      |     fprintf('%s -- Copyright %s Nexteer',NxtrConf,first)
      | else
      |     fprintf('%s -- %s%s- %s Nexteer',NxtrConf,char(169),first,last)
      | end
  Max_f32 : NxtrMax/Max_f32  SFunctionSpec=single y1 = Max_f32(single u1, single u2)
      settings: AttributesFormatString=%<Name>
  Product1 : Product  RndMeth=Zero
  Sign_s08_f32 : NxtrSign/Sign_s08_f32  SFunctionSpec=int8 y1 = Sign_s08_f32(single u1)
  Out : Outport
  wires:
  DampgCmdScad/1 -> Abslt_f32_f32/1
  Abslt_f32_f32/1 -> Max_f32/1
  Abslt_f32_f1/1 -> Max_f32/2
  Max_f32/1 -> Product1/1
  Sign_s08_f32/1 -> Product1/2
  CustomDmpg/1 -> Abslt_f32_f1/1
  CalcdMotVelCrf/1 -> Sign_s08_f32/1
  Product1/1 -> Out/1

== system SF003A_Dampg/Dampg/DampgPer1/CmdDiChk/Zero_Command ==
  Action Port : ActionPort  ActionType=then
  Constant1 : Constant  RequirementInfo={} %GIDa_b06efe7e_48c8_49f6_a833_04aad4eae373  Value=0  OutDataTypeStr=single
  CopyRight2 : Subsystem  Description=|  mask(Copyright Information){none=on}
      | Copyright info block.                                               
      |                                                                     
      | Place copyright information at the top of every subsystem in design.
      mask prompts: none "No parameters"
      mask help: Place copyright information at the top of every subsystem in design.
      mask Display:
      | NxtrConf = 'Nexteer Confidential';
      | 
      | sys = bdroot; %handle for the current model ("system")
      | first = get_param(sys,'Created');
      | if(isempty(first))
      |     first = datestr(now,'yyyy');
      | else
      |     first = first(end-3:end);  %year is last four digits
      | end
      | 
      | last = get_param(sys,'LastModifiedDate');
      | if isempty(last)
      |     last = datestr(now,'yyyy');
      | else
      |     last = last(end-3:end);
      | end
      | 
      | if strcmp(first,last)
      |     fprintf('%s -- Copyright %s Nexteer',NxtrConf,first)
      | else
      |     fprintf('%s -- %s%s- %s Nexteer',NxtrConf,char(169),first,last)
      | end
  Out : Outport
  wires:
  Constant1/1 -> Out/1

== system SF003A_Dampg/Dampg/DampgPer1/FltInj - Sim/CopyRight2 ==

== system SF003A_Dampg/Dampg/DampgPer1/HydPwrSteerDampgCmd/CopyRight2 ==

== system SF003A_Dampg/Dampg/DampgPer1/MotVelDampgCmd/CopyRight2 ==

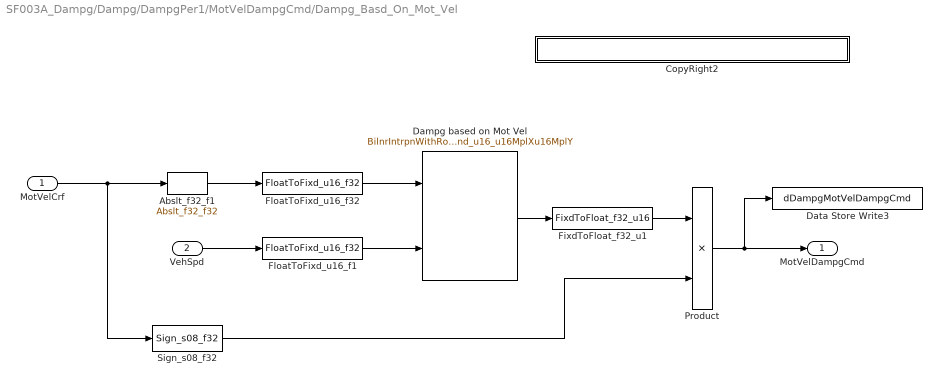
== system SF003A_Dampg/Dampg/DampgPer1/MotVelDampgCmd/Dampg_Basd_On_Mot_Vel ==
  MotVelCrf : Inport
  VehSpd : Inport  Port=2
  Abslt_f32_f1 : NxtrAbslt/Abslt_f32_f32  SFunctionSpec=single y1 = Abslt_f32_f32(single u1)
      settings: AttributesFormatString=%<Name>
  CopyRight2 : Subsystem  Description=|  mask(Copyright Information){none=on}
      | Copyright info block.                                               
      |                                                                     
      | Place copyright information at the top of every subsystem in design.
      mask prompts: none "No parameters"
      mask help: Place copyright information at the top of every subsystem in design.
      mask Display:
      | NxtrConf = 'Nexteer Confidential';
      | 
      | sys = bdroot; %handle for the current model ("system")
      | first = get_param(sys,'Created');
      | if(isempty(first))
      |     first = datestr(now,'yyyy');
      | else
      |     first = first(end-3:end);  %year is last four digits
      | end
      | 
      | last = get_param(sys,'LastModifiedDate');
      | if isempty(last)
      |     last = datestr(now,'yyyy');
      | else
      |     last = last(end-3:end);
      | end
      | 
      | if strcmp(first,last)
      |     fprintf('%s -- Copyright %s Nexteer',NxtrConf,first)
      | else
      |     fprintf('%s -- %s%s- %s Nexteer',NxtrConf,char(169),first,last)
      | end
  Dampg based on Mot Vel : BilnrIntrpnMplX/BilnrIntrpnWithRound_u16_u16MplXu16MplY  MplXTbl=DampgMotVelX  MplYTbl=DampgMotVelY  BilnrSelnTbl=SysGlbPrmVehSpdBilnrSeln
      settings: AttributesFormatString=Bilnr ( u16MplX , u16MplY )
  Data Store Write3 : DataStoreWrite  DataStoreName=dDampgMotVelDampgCmd
  FixdToFloat_f32_u1 : FixdToFloat/FixdToFloat_f32_u16  Param1=11
  FloatToFixd_u16_f1 : FloatToFixd/FloatToFixd_u16_f32  Param1=7
  FloatToFixd_u16_f32 : FloatToFixd/FloatToFixd_u16_f32  Param1=4
  Product : Product  RndMeth=Zero
  Sign_s08_f32 : NxtrSign/Sign_s08_f32  SFunctionSpec=int8 y1 = Sign_s08_f32(single u1)
  MotVelDampgCmd : Outport
  wires:
  Sign_s08_f32/1 -> Product/2
  MotVelCrf/1 -> Abslt_f32_f1/1, Sign_s08_f32/1
  FloatToFixd_u16_f32/1 -> Dampg based on Mot Vel/1
  FloatToFixd_u16_f1/1 -> Dampg based on Mot Vel/2
  Dampg based on Mot Vel/1 -> FixdToFloat_f32_u1/1
  Abslt_f32_f1/1 -> FloatToFixd_u16_f32/1
  VehSpd/1 -> FloatToFixd_u16_f1/1
  Product/1 -> Data Store Write3/1, MotVelDampgCmd/1
  FixdToFloat_f32_u1/1 -> Product/1

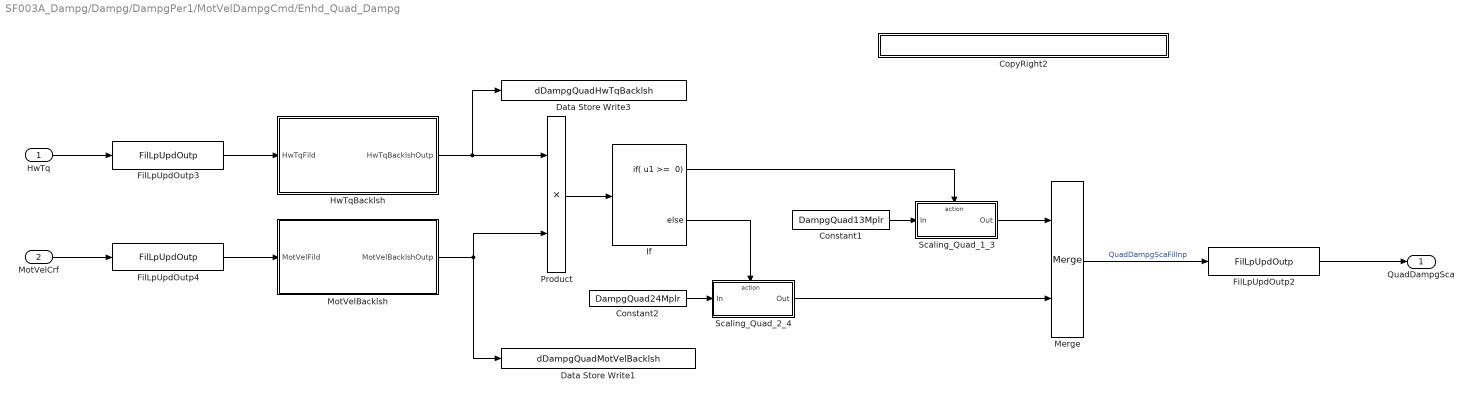
== system SF003A_Dampg/Dampg/DampgPer1/MotVelDampgCmd/Enhd_Quad_Dampg  ==
  HwTq : Inport
  MotVelCrf : Inport  Port=2
  Constant1 : Constant  RequirementInfo={} %GIDa_5b902024_3e8c_4494_84c3_91dcbfea766a  Value=DampgQuad13Mplr  OutDataTypeStr=single
  Constant2 : Constant  RequirementInfo={} %GIDa_587e475f_d2d7_438f_8480_63dc4e95efa6  Value=DampgQuad24Mplr  OutDataTypeStr=single
  CopyRight2 : Subsystem  Description=|  mask(Copyright Information){none=on}
      | Copyright info block.                                               
      |                                                                     
      | Place copyright information at the top of every subsystem in design.
      mask prompts: none "No parameters"
      mask help: Place copyright information at the top of every subsystem in design.
      mask Display:
      | NxtrConf = 'Nexteer Confidential';
      | 
      | sys = bdroot; %handle for the current model ("system")
      | first = get_param(sys,'Created');
      | if(isempty(first))
      |     first = datestr(now,'yyyy');
      | else
      |     first = first(end-3:end);  %year is last four digits
      | end
      | 
      | last = get_param(sys,'LastModifiedDate');
      | if isempty(last)
      |     last = datestr(now,'yyyy');
      | else
      |     last = last(end-3:end);
      | end
      | 
      | if strcmp(first,last)
      |     fprintf('%s -- Copyright %s Nexteer',NxtrConf,first)
      | else
      |     fprintf('%s -- %s%s- %s Nexteer',NxtrConf,char(169),first,last)
      | end
  Data Store Write1 : DataStoreWrite  DataStoreName=dDampgQuadMotVelBacklsh
  Data Store Write3 : DataStoreWrite  DataStoreName=dDampgQuadHwTqBacklsh
  FilLpUpdOutp2 : Fil/FilLpUpdOutp  StVar=QuadDampgScaLpFil
      settings: AttributesFormatString=StVar: %<StVar>
  FilLpUpdOutp3 : Fil/FilLpUpdOutp  StVar=QuadDampgHwTqLpFil
      settings: AttributesFormatString=StVar: %<StVar>
  FilLpUpdOutp4 : Fil/FilLpUpdOutp  StVar=QuadDampgMotVelLpFil
      settings: AttributesFormatString=StVar: %<StVar>
  HwTqBacklsh : Subsystem
  If : If  IfExpression="u1 >=  0"
  Merge : Merge
  MotVelBacklsh : Subsystem
  Product : Product  RndMeth=Zero
  Scaling_Quad_1_3 : Subsystem  RequirementInfo={} %GIDa_485cad3f_31a8_4856_95a7_16cb3f5dc668  TreatAsAtomicUnit=on
  Scaling_Quad_2_4 : Subsystem  RequirementInfo={} %GIDa_b28b5c6d_494b_445a_b5ee_da8ce8308b9a  TreatAsAtomicUnit=on
  QuadDampgSca : Outport
  wires:
  MotVelCrf/1 -> FilLpUpdOutp4/1
  HwTq/1 -> FilLpUpdOutp3/1
  MotVelBacklsh/1(MotVelBacklshOutp) -> Data Store Write1/1, Product/2
  Product/1 -> If/1
  If/1 -> Scaling_Quad_1_3/Action
  If/2 -> Scaling_Quad_2_4/Action
  Scaling_Quad_1_3/1(Out) -> Merge/1
  Merge/1 -> FilLpUpdOutp2/1  "QuadDampgScaFilInp"
  FilLpUpdOutp2/1 -> QuadDampgSca/1
  Constant1/1 -> Scaling_Quad_1_3/1(In)
  Constant2/1 -> Scaling_Quad_2_4/1(In)
  Scaling_Quad_2_4/1(Out) -> Merge/2
  FilLpUpdOutp4/1 -> MotVelBacklsh/1(MotVelFild)
  HwTqBacklsh/1(HwTqBacklshOutp) -> Data Store Write3/1, Product/1
  FilLpUpdOutp3/1 -> HwTqBacklsh/1(HwTqFild)

== system SF003A_Dampg/Dampg/DampgPer1/CmdDiChk/DmpgCmdChk/CopyRight2 ==

== system SF003A_Dampg/Dampg/DampgPer1/CmdDiChk/Zero_Command/CopyRight2 ==

== system SF003A_Dampg/Dampg/DampgPer1/MotVelDampgCmd/Dampg_Basd_On_Mot_Vel/CopyRight2 ==

== system SF003A_Dampg/Dampg/DampgPer1/MotVelDampgCmd/Enhd_Quad_Dampg /CopyRight2 ==

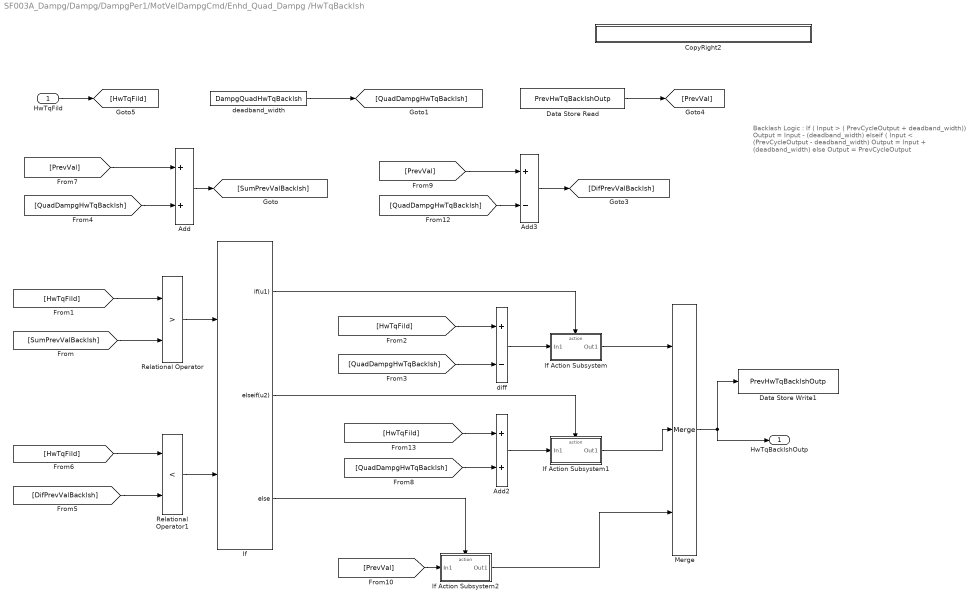
== system SF003A_Dampg/Dampg/DampgPer1/MotVelDampgCmd/Enhd_Quad_Dampg /HwTqBacklsh ==
  note: Backlash Logic :
      | If ( Input > ( PrevCycleOutput + deadband_width))
      | 	Output = Input - (deadband_width)
      | elseif ( Input < (PrevCycleOutput - deadband_width)
      | 	Output = Input + (deadband_width)
      | else
      | 	Output = PrevCycleOutput
  HwTqFild : Inport
  Add : Sum
  Add2 : Sum
  Add3 : Sum  Inputs=+-
  CopyRight2 : Subsystem  Description=|  mask(Copyright Information){none=on}
      | Copyright info block.                                               
      |                                                                     
      | Place copyright information at the top of every subsystem in design.
      mask prompts: none "No parameters"
      mask help: Place copyright information at the top of every subsystem in design.
      mask Display:
      | NxtrConf = 'Nexteer Confidential';
      | 
      | sys = bdroot; %handle for the current model ("system")
      | first = get_param(sys,'Created');
      | if(isempty(first))
      |     first = datestr(now,'yyyy');
      | else
      |     first = first(end-3:end);  %year is last four digits
      | end
      | 
      | last = get_param(sys,'LastModifiedDate');
      | if isempty(last)
      |     last = datestr(now,'yyyy');
      | else
      |     last = last(end-3:end);
      | end
      | 
      | if strcmp(first,last)
      |     fprintf('%s -- Copyright %s Nexteer',NxtrConf,first)
      | else
      |     fprintf('%s -- %s%s- %s Nexteer',NxtrConf,char(169),first,last)
      | end
  Data Store Read : DataStoreRead  DataStoreName=PrevHwTqBacklshOutp
  Data Store Write1 : DataStoreWrite  DataStoreName=PrevHwTqBacklshOutp
  If : If  NumInputs=2  IfExpression=u1  ElseIfExpressions=u2
  If Action Subsystem : Subsystem  TreatAsAtomicUnit=on
  If Action Subsystem1 : Subsystem  TreatAsAtomicUnit=on
  If Action Subsystem2 : Subsystem  TreatAsAtomicUnit=on
  Merge : Merge  Inputs=3
  Relational Operator : RelationalOperator  Operator=>  OutDataTypeStr=boolean
  Relational Operator1 : RelationalOperator  Operator=<  OutDataTypeStr=boolean
  deadband_width : Constant  Value=DampgQuadHwTqBacklsh  OutDataTypeStr=single
  diff : Sum  Inputs=+-
  HwTqBacklshOutp : Outport
  wires:
  Relational Operator/1 -> If/1
  [SumPrevValBacklsh] -> Relational Operator/2
  [HwTqFild] -> Relational Operator/1
  diff/1 -> If Action Subsystem/1(In1)
  [HwTqFild] -> diff/1
  [QuadDampgHwTqBacklsh] -> diff/2
  If/1 -> If Action Subsystem/Action
  [HwTqFild] -> Relational Operator1/1
  [DifPrevValBacklsh] -> Relational Operator1/2
  Relational Operator1/1 -> If/2
  [HwTqFild] -> Add2/1
  [QuadDampgHwTqBacklsh] -> Add2/2
  Add2/1 -> If Action Subsystem1/1(In1)
  If/2 -> If Action Subsystem1/Action
  [PrevVal] -> If Action Subsystem2/1(In1)
  If/3 -> If Action Subsystem2/Action
  If Action Subsystem1/1(Out1) -> Merge/2
  If Action Subsystem2/1(Out1) -> Merge/3
  If Action Subsystem/1(Out1) -> Merge/1
  Merge/1 -> HwTqBacklshOutp/1, Data Store Write1/1
  deadband_width/1 -> [QuadDampgHwTqBacklsh]
  Add/1 -> [SumPrevValBacklsh]
  [PrevVal] -> Add/1
  [QuadDampgHwTqBacklsh] -> Add/2
  Add3/1 -> [DifPrevValBacklsh]
  [PrevVal] -> Add3/1
  [QuadDampgHwTqBacklsh] -> Add3/2
  Data Store Read/1 -> [PrevVal]
  HwTqFild/1 -> [HwTqFild]

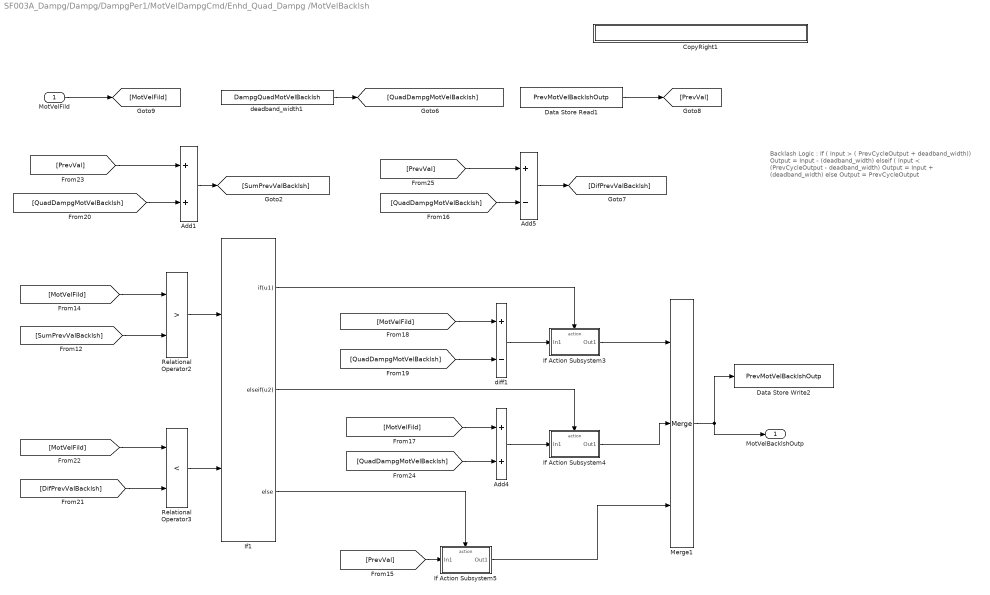
== system SF003A_Dampg/Dampg/DampgPer1/MotVelDampgCmd/Enhd_Quad_Dampg /MotVelBacklsh ==
  note: Backlash Logic :
      | If ( Input > ( PrevCycleOutput + deadband_width))
      | 	Output = Input - (deadband_width)
      | elseif ( Input < (PrevCycleOutput - deadband_width)
      | 	Output = Input + (deadband_width)
      | else
      | 	Output = PrevCycleOutput
  MotVelFild : Inport
  Add1 : Sum
  Add4 : Sum
  Add5 : Sum  Inputs=+-
  CopyRight1 : Subsystem  Description=|  mask(Copyright Information){none=on}
      | Copyright info block.                                               
      |                                                                     
      | Place copyright information at the top of every subsystem in design.
      mask prompts: none "No parameters"
      mask help: Place copyright information at the top of every subsystem in design.
      mask Display:
      | NxtrConf = 'Nexteer Confidential';
      | 
      | sys = bdroot; %handle for the current model ("system")
      | first = get_param(sys,'Created');
      | if(isempty(first))
      |     first = datestr(now,'yyyy');
      | else
      |     first = first(end-3:end);  %year is last four digits
      | end
      | 
      | last = get_param(sys,'LastModifiedDate');
      | if isempty(last)
      |     last = datestr(now,'yyyy');
      | else
      |     last = last(end-3:end);
      | end
      | 
      | if strcmp(first,last)
      |     fprintf('%s -- Copyright %s Nexteer',NxtrConf,first)
      | else
      |     fprintf('%s -- %s%s- %s Nexteer',NxtrConf,char(169),first,last)
      | end
  Data Store Read1 : DataStoreRead  DataStoreName=PrevMotVelBacklshOutp
  Data Store Write2 : DataStoreWrite  DataStoreName=PrevMotVelBacklshOutp
  If Action Subsystem3 : Subsystem  TreatAsAtomicUnit=on
  If Action Subsystem4 : Subsystem  TreatAsAtomicUnit=on
  If Action Subsystem5 : Subsystem  TreatAsAtomicUnit=on
  If1 : If  NumInputs=2  IfExpression=u1  ElseIfExpressions=u2
  Merge1 : Merge  Inputs=3
  Relational Operator2 : RelationalOperator  Operator=>  OutDataTypeStr=boolean
  Relational Operator3 : RelationalOperator  Operator=<  OutDataTypeStr=boolean
  deadband_width1 : Constant  Value=DampgQuadMotVelBacklsh  OutDataTypeStr=single
  diff1 : Sum  Inputs=+-
  MotVelBacklshOutp : Outport
  wires:
  Relational Operator2/1 -> If1/1
  [SumPrevValBacklsh] -> Relational Operator2/2
  [MotVelFild] -> Relational Operator2/1
  diff1/1 -> If Action Subsystem3/1(In1)
  [MotVelFild] -> diff1/1
  [QuadDampgMotVelBacklsh] -> diff1/2
  If1/1 -> If Action Subsystem3/Action
  [MotVelFild] -> Relational Operator3/1
  [DifPrevValBacklsh] -> Relational Operator3/2
  Relational Operator3/1 -> If1/2
  [MotVelFild] -> Add4/1
  [QuadDampgMotVelBacklsh] -> Add4/2
  Add4/1 -> If Action Subsystem4/1(In1)
  If1/2 -> If Action Subsystem4/Action
  [PrevVal] -> If Action Subsystem5/1(In1)
  If1/3 -> If Action Subsystem5/Action
  If Action Subsystem4/1(Out1) -> Merge1/2
  If Action Subsystem5/1(Out1) -> Merge1/3
  If Action Subsystem3/1(Out1) -> Merge1/1
  Merge1/1 -> MotVelBacklshOutp/1, Data Store Write2/1
  deadband_width1/1 -> [QuadDampgMotVelBacklsh]
  Add1/1 -> [SumPrevValBacklsh]
  [PrevVal] -> Add1/1
  [QuadDampgMotVelBacklsh] -> Add1/2
  Add5/1 -> [DifPrevValBacklsh]
  [PrevVal] -> Add5/1
  [QuadDampgMotVelBacklsh] -> Add5/2
  Data Store Read1/1 -> [PrevVal]
  MotVelFild/1 -> [MotVelFild]

== system SF003A_Dampg/Dampg/DampgPer1/MotVelDampgCmd/Enhd_Quad_Dampg /Scaling_Quad_1_3 ==
  In : Inport
  Action Port : ActionPort  ActionType=then
  Out : Outport
  wires:
  In/1 -> Out/1

== system SF003A_Dampg/Dampg/DampgPer1/MotVelDampgCmd/Enhd_Quad_Dampg /Scaling_Quad_2_4 ==
  In : Inport
  Action Port : ActionPort  ActionType=else
  Out : Outport
  wires:
  In/1 -> Out/1

== system SF003A_Dampg/Dampg/DampgPer1/MotVelDampgCmd/Enhd_Quad_Dampg /HwTqBacklsh/CopyRight2 ==

== system SF003A_Dampg/Dampg/DampgPer1/MotVelDampgCmd/Enhd_Quad_Dampg /HwTqBacklsh/If Action Subsystem ==
  In1 : Inport
  Action Port : ActionPort  ActionType=then
  Out1 : Outport
  wires:
  In1/1 -> Out1/1

== system SF003A_Dampg/Dampg/DampgPer1/MotVelDampgCmd/Enhd_Quad_Dampg /HwTqBacklsh/If Action Subsystem1 ==
  In1 : Inport
  Action Port : ActionPort  ActionType=elseif
  Out1 : Outport
  wires:
  In1/1 -> Out1/1

== system SF003A_Dampg/Dampg/DampgPer1/MotVelDampgCmd/Enhd_Quad_Dampg /HwTqBacklsh/If Action Subsystem2 ==
  In1 : Inport
  Action Port : ActionPort  ActionType=else
  Out1 : Outport
  wires:
  In1/1 -> Out1/1

== system SF003A_Dampg/Dampg/DampgPer1/MotVelDampgCmd/Enhd_Quad_Dampg /MotVelBacklsh/CopyRight1 ==

== system SF003A_Dampg/Dampg/DampgPer1/MotVelDampgCmd/Enhd_Quad_Dampg /MotVelBacklsh/If Action Subsystem3 ==
  In1 : Inport
  Action Port : ActionPort  ActionType=then
  Out1 : Outport
  wires:
  In1/1 -> Out1/1

== system SF003A_Dampg/Dampg/DampgPer1/MotVelDampgCmd/Enhd_Quad_Dampg /MotVelBacklsh/If Action Subsystem4 ==
  In1 : Inport
  Action Port : ActionPort  ActionType=elseif
  Out1 : Outport
  wires:
  In1/1 -> Out1/1

== system SF003A_Dampg/Dampg/DampgPer1/MotVelDampgCmd/Enhd_Quad_Dampg /MotVelBacklsh/If Action Subsystem5 ==
  In1 : Inport
  Action Port : ActionPort  ActionType=else
  Out1 : Outport
  wires:
  In1/1 -> Out1/1
